simulink model "valve_ports"  (R2020b)
settings: Solver=VariableStepAuto  StartTime=0.0  StopTime=inf  RelTol=1e-3
undefined symbols (not defined in the file or in its folder): daq
libraries: daqlib x2, dspfdesign x1, dspstat3 x1, eeGeneralControl x1, pid_lib x1
settings Model: Creator=SIRIL D. TEJA  LastModifiedBy=Siril TD

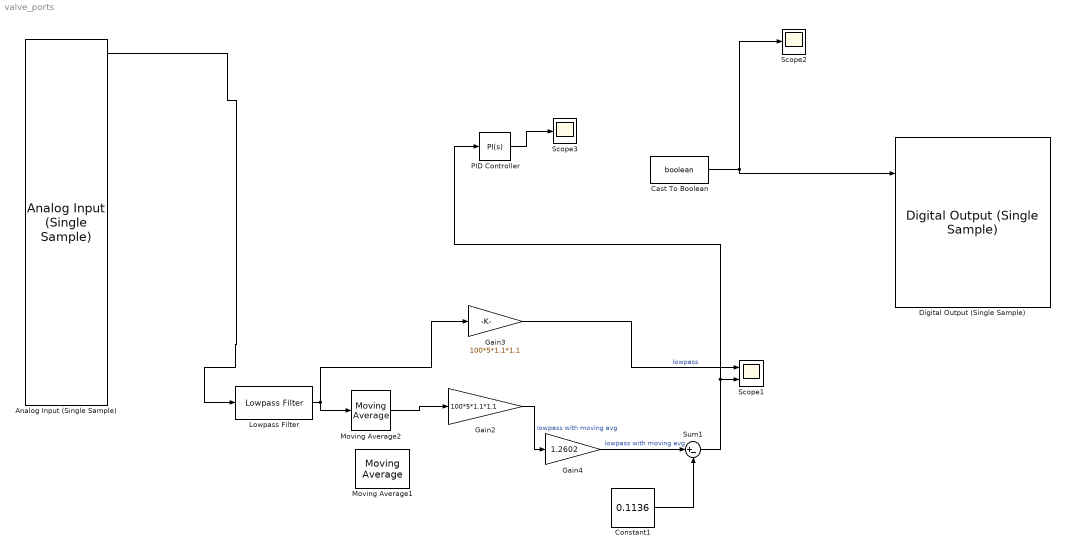
== system valve_ports ==
  Analog Input (Single Sample) : daqlib/Analog Input (Single Sample)  DeviceMenu=ni cDAQ1 (cDAQ-9178)  Device=ni cDAQ1 (cDAQ-9178)  ModuleInfo=cDAQ1Mod5(NI 9205)  ObjConstructor=daq.createSession('ni')  BlockSampleTime=1  NChannelsSelected=32  Channels=1$ai0$$cDAQ1Mod5$1$4$3$1$#1$ai1$$cDAQ1Mod5$1$4$3$1$#1$ai2$$cDAQ1Mod5$1$4$3$1$#1$ai3$$cDAQ1Mod5$1$4$3$1$#1$ai4$$cDAQ1Mod5$1$4$3$1$#1$ai5$$cDAQ1Mod5$1$4$3$1$#1$ai6$$cDAQ1Mod5$1$4$3$1$#1$ai7$$cDAQ1Mod5$1$4$3$1$#1$ai8$$cDAQ1Mod5$1$4$1$1$#1$ai9$$cDAQ1Mod5$1$4$1$1$#1$ai10$$cDAQ1Mod5$1$4$1$1$#1$ai11$$cDAQ1Mod5$1$4$1$1$#1$ai12$$cDAQ1Mod5$1$4$1$1$#1$ai13$$cDAQ1Mod5$1$4$1$1$#1$ai14$$cDAQ1Mod5$1$4$1$1$#1$ai15$$cDAQ1Mod5$1$4$1$1$#1$ai16$$cDAQ1Mod5$1$4$3$1$#1$ai17$$cDAQ1Mod5$1$4$3$1$#1$ai18$$cDAQ1Mod5$1$4$3$1$#1$ai19$$cDAQ1Mod5$1$4$3$1$#1$ai20$$cDAQ1Mod5$1$4$3$1$#1$ai21$$cDAQ1Mod5$1$4$3$1$#1$ai22$$cDAQ1Mod5$1$4$3$1$#1$ai23$$cDAQ1Mod5$1$4$3$1$#1$ai24$$cDAQ1Mod5$1$4$1$1$#1$ai25$$cDAQ1Mod5$1$4$1$1$#1$ai26$$cDAQ1Mod5$1$4$1$1$#1$ai27$$cDAQ1Mod5$1$4$1$1$#1$ai28$$cDAQ1Mod5$1$4$1$1$#1$ai29$$cDAQ1Mod5$1$4$1$1$#1$ai30$$cDAQ1Mod5$1$4$1$1$#1$ai31$$cDAQ1Mod5$1$4$1$1$#  NPorts=1 per channel  OutputTimestamp=off
      settings: SourceProductBaseCode=DA
  Cast To Boolean : DataTypeConversion  OutDataTypeStr=boolean
  Constant1 : Constant  Value=0.1136
  Digital Output (Single Sample) : daqlib/Digital Output (Single Sample)  DeviceMenu=ni cDAQ1 (cDAQ-9178)  Device=ni cDAQ1 (cDAQ-9178)  ModuleInfo=cDAQ1Mod1(NI 9485)  ObjConstructor=daq.createSession('ni')  BlockSampleTime=1  IsDigitalInput=off  NLinesSelected=8  Lines=1$port0/line0$$cDAQ1Mod1$#1$port0/line1$$cDAQ1Mod1$#1$port0/line2$$cDAQ1Mod1$#1$port0/line3$$cDAQ1Mod1$#1$port0/line4$$cDAQ1Mod1$#1$port0/line5$$cDAQ1Mod1$#1$port0/line6$$cDAQ1Mod1$#1$port0/line7$$cDAQ1Mod1$#  NPorts=1 per line
      settings: SourceProductBaseCode=DA
  Gain2 : Gain  Gain=100*5*1.1*1.1
  Gain3 : Gain  Gain=100*5*1.1*1.1
  Gain4 : Gain  Gain=1.2602
  Lowpass Filter : dspfdesign/Lowpass Filter  FilterType=FIR  DesignForMinimumOrder=on  FilterOrder=50  PassbandFrequency=8e3  StopbandFrequency=12e3  PassbandRipple=0.1  StopbandAttenuation=80  InheritSampleRate=off  SampleRate=41500  SimulateUsing=Code generation  roundingMode=Floor  coeffsDataTypeStr=fixdt(1,16)
  Moving Average2 : dspstat3/Moving Average  Method=Exponential weighting  ForgettingFactorPort=off  SpecifyWindowLength=on  WindowLength=4  ForgettingFactor=0.99  SimulateUsing=Code generation
  Moving Average1 : eeGeneralControl/Moving Average  VariantControl=Variant1  LabelModeActiveChoice=Discrete  f=500  x0=0  Ts=-1
      settings: SourceProductBaseCode=PS
  PID Controller : pid_lib/PID Controller  Controller=PI  Form=Ideal  TimeDomain=Continuous-time  UseExternalTs=off  SampleTime=-1  IntegratorMethod=Forward Euler  FilterMethod=Forward Euler  ControllerParametersSource=internal  P=1  I=.5  D=0  UseFilter=on  N=100  TunerSelectOption=Transfer Function Based (PID Tuner App)  InitialConditionSource=internal  InitialConditionForIntegrator=0  InitialConditionForFilter=0  DifferentiatorICPrevScaledInput=0  ExternalReset=none  TrackingMode=off  Kt=1  LimitOutput=off  SatLimitsSource=internal  UpperSaturationLimit=inf  LowerSaturationLimit=-inf  LinearizeAsGain=on  AntiWindupMode=none  Kb=1  POutMin=[]  POutMax=[]  IOutMin=[]  IOutMax=[]  DOutMin=[]  DOutMax=[]  NOutMin=[]  NOutMax=[]  SumOutMin=[]  SumOutMax=[]  SaturationOutMin=[]  SaturationOutMax=[]  PParamMin=[]  PParamMax=[]  IParamMin=[]  IParamMax=[]  DParamMin=[]  DParamMax=[]  NParamMin=[]  NParamMax=[]  KbParamMin=[]  KbParamMax=[]  KtParamMin=[]  KtParamMax=[]  KbOutMin=[]  KbOutMax=[]  KtOutMin=[]  KtOutMax=[]  IntegratorOutMin=[]  IntegratorOutMax=[]  FilterOutMin=[]  FilterOutMax=[]  SumI1OutMin=[]  SumI1OutMax=[]  SumI2OutMin=[]  SumI2OutMax=[]  SumI3OutMin=[]  SumI3OutMax=[]  SumI4OutMin=[]  SumI4OutMax=[]  SumDOutMin=[]  SumDOutMax=[]  DifferentiatorOutMin=[]  DifferentiatorOutMax=[]  FilterDiffOutCoefMin=[]  FilterDiffOutCoefMax=[]  ReciprocalOutMin=[]  ReciprocalOutMax=[]  SumDenOutMin=[]  SumDenOutMax=[]  SumNumOutMin=[]  SumNumOutMax=[]  DivideOutMin=[]  DivideOutMax=[]  UdiffTsProdOutMin=[]  UdiffTsProdOutMax=[]  NTsProdOutMin=[]  NTsProdOutMax=[]  UintegralTsProdOutMin=[]  UintegralTsProdOutMax=[]  UngainTsProdOutMin=[]  UngainTsProdOutMax=[]  IntegratorContinuousStateAttributes=''  IntegratorStateMustResolveToSignalObject=off  IntegratorRTWStateStorageClass=Auto  FilterContinuousStateAttributes=''  FilterStateMustResolveToSignalObject=off  FilterRTWStateStorageClass=Auto  ParallelPVariant=Passthrough  IdealPVariant=InternalParameters  IVariant=InternalParameters  DVariant=Disabled  IntegratorVariant=Continuous  SatVariant=Disabled  AWVariant=Passthrough  PCopyVariant=Disabled  TRVariant=Disabled  FdbkBlocksVariant=Forward  IdealPFdbkVariant=Disabled  SatFdbkVariant=Disabled  DerivativeFilterVariant=Disabled  NVariant=Disabled  NCopyVariant=Disabled_SignalSpec  FilterICVariant=Disabled  IntegratorICVariant=InternalICs  ExternalResetVariant=Disabled  TRSumVariant=Passthrough  SumFdbkVariant=Disabled  SumVariant=Sum_PI  TsampFilterVariant=InternalTs  TsampNgainVariant=Passthrough  TsampIntegralVariant=Passthrough  ExternalSaturationOutDataTypeStr=Inherit: Same as second input
  Scope1 : Scope  NumInputPorts=2
  Scope2 : Scope
  Scope3 : Scope
  Sum1 : Sum  Inputs=|+-
  wires:
  Cast To Boolean/1 -> Scope2/1, Digital Output (Single Sample)/2
  Analog Input (Single Sample)/2 -> Lowpass Filter/1
  Gain2/1 -> Gain4/1  "lowpass with moving avg"
  Lowpass Filter/1 -> Gain3/1, Moving Average2/1
  Gain3/1 -> Scope1/1  "lowpass"
  Moving Average2/1 -> Gain2/1
  Constant1/1 -> Sum1/2
  Gain4/1 -> Sum1/1  "lowpass with moving avg"
  Sum1/1 -> PID Controller/1, Scope1/2
  PID Controller/1 -> Scope3/1
